simulink model "WL_3_0"  (R2025a)
settings: Solver=ode4  StartTime=0.0  StopTime=T_sim  FixedStep=Dt_sim  RelTol=1e-3
InitFcn:
  | % --- AVVIO AUTOMATICO PYTHON SERVER CON POP-UP (METODO FILE ROBUSTO) ---
  | fprintf('[Simulink] Preparazione simulazione...\n');
  | 
  | % 1. Pop-up per la Raffica
  | scelta_gust = questdlg('Vuoi includere la raffica (gust_H40.gust)?', ...
  |     'Configurazione Raffica', 'Si', 'No', 'No');
  | if isempty(scelta_gust), scelta_gust = 'No'; end
  | 
  | % 2. Pop-up per il Video
  | scelta_video = questdlg('Vuoi generare il video MP4 a fine simulazione?', ...
  |     'Configurazione Video', 'Si', 'No', 'No');
  | if isempty(scelta_video), scelta_video = 'No'; end
  | 
  | % --- PERCORSO ASSOLUTO ---
  | % Definiamo subito la cartella così MATLAB e WSL salvano e leggono dallo stesso posto
  | percorso = '/home/lpmatteo/Internship_INCARBONE_2026/LQR_first_controller_study/LQR_WL_simulation';
  | file_inputs = fullfile(percorso, 'python_inputs.txt');
  | 
  | % --- CREAZIONE FILE DI INPUT ---
  | fid = fopen(file_inputs, 'w');
  | fprintf(fid, '1\n'); % Scelta controller: 1 (LQI)
  | 
  | if strcmp(scelta_gust, 'Si')
  |     fprintf(fid, 's\n');
  | else
  |     fprintf(fid, 'n\n');
  | end
  | 
  | if strcmp(scelta_video, 'Si')
  |     % Se vogliamo il video, precompiliamo anche formato (mp4), qualità (high)
  |     % e la "Y" finale per far partire il render ASWING in automatico.
  |     fprintf(fid, 's\ngif\nmedium\nY\n');
  | else
  |     fprintf(fid, 'n\n');
  | end
  | fclose(fid);
  | 
  | % --- AVVIO DEL SERVER WSL ---
  | % Diciamo a Python di prendere le risposte direttamente dal file appena creato
  | cmd_wsl = sprintf('start "WingLoop Python Server" wsl -e bash -ic "cd %s && conda activate WINGLOOP && python3 controller_wingloop.py < python_inputs.txt; exec bash"', percorso);
  | 
  | system(cmd_wsl);
values from neighbouring files (symbols this model uses):
  u_trim = [0, F2ref, F3ref, 0, E2ref, E2ref]    [WL_main.m]
undefined symbols (not defined in the file or in its folder): FullModel, idx, K_z, matrices, ref_vec
libraries: cstblocks x1
settings Model: SimulationMode=accelerator  Creator=lpmat  LastModifiedBy=lpmat

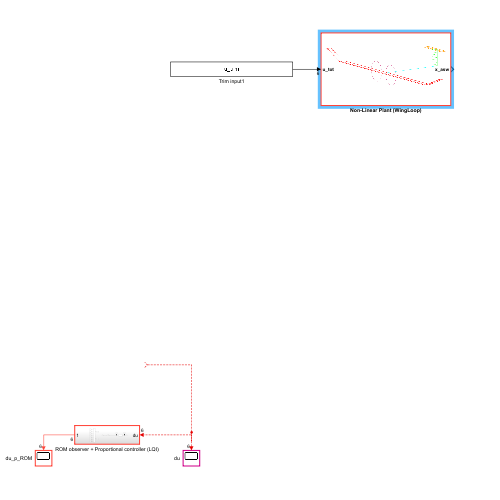
[thumbnail: Simulink's stored preview of the top-level diagram]
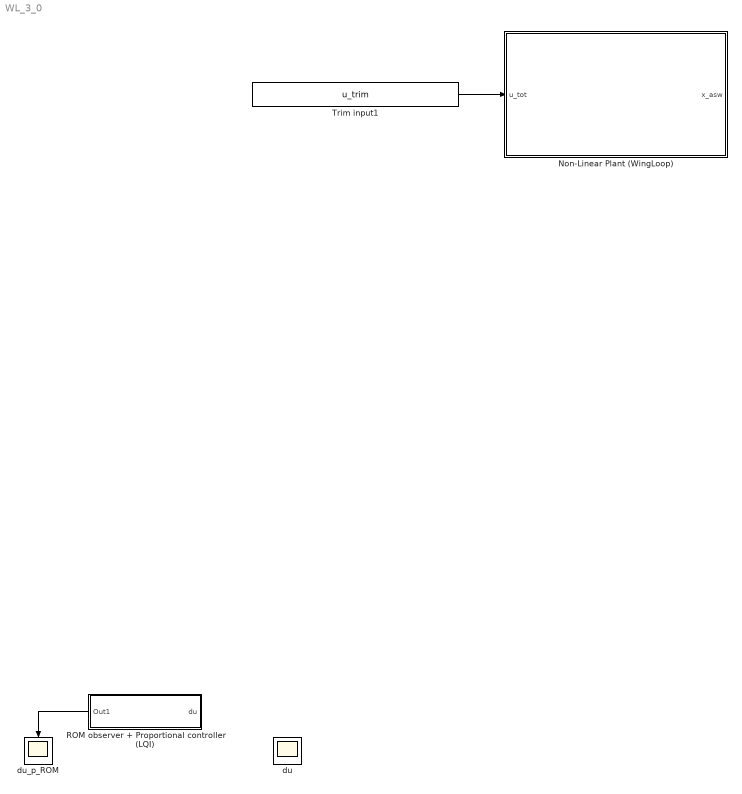
== system WL_3_0 ==
  Non-Linear Plant (WingLoop) : Subsystem
      mask Display: image('Screenshot 2026-03-18 123158.png');
  ROM observer + Proportional controller (LQI) : Subsystem
  Trim input1 : Constant  Value=u_trim
  du : Scope
      settings: ActiveDisplayYMinimum=-1  ActiveDisplayYMaximum=1  DataLoggingVariableName=ScopeData15
  du_p_ROM : Scope
      settings: ActiveDisplayYMinimum=-1  ActiveDisplayYMaximum=1  DataLoggingVariableName=ScopeData10
  wires:
  Trim input1/1 -> Non-Linear Plant (WingLoop)/1(u_tot)
  ROM observer + Proportional controller (LQI)/1(Out1) -> du_p_ROM/1
  ? -> ROM observer + Proportional controller (LQI)/1(du), du/1

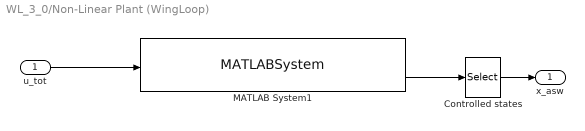
== system WL_3_0/Non-Linear Plant (WingLoop) ==
  u_tot : Inport
  Controlled states : Selector  InputPortWidth=1888  IndexOptions=Index vector (dialog)  Indices=[1:1882]  OutputSizes=1
  MATLAB System1 : MATLABSystem  System=AswingPlant  ServerHost=localhost  ServerPort=5005  NumModalStates=ROM.n_modal  NumPhysicalStates=FullModel.n_orig+ FullModel.n_in  SimulateUsing=Interpreted execution
      mask Type: AswingPlant
  x_asw : Outport
  wires:
  MATLAB System1/2 -> Controlled states/1
  u_tot/1 -> MATLAB System1/1
  Controlled states/1 -> x_asw/1

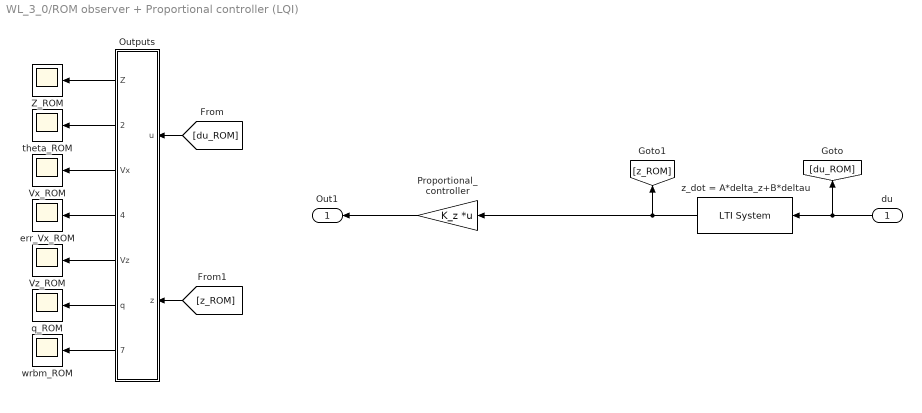
== system WL_3_0/ROM observer + Proportional controller (LQI) ==
  du : Inport
  Outputs : Subsystem
  Proportional_controller : Gain  Gain=K_z  Multiplication=Matrix(K*u)
  Vx_ROM : Scope
      settings: ActiveDisplayYMinimum=-29.75997799121388  ActiveDisplayYMaximum=-29.616858798151441  DataLoggingVariableName=ScopeData28
  Vz_ROM : Scope
      settings: ActiveDisplayYMinimum=-2.6148202510273633  ActiveDisplayYMaximum=-2.6136511943302931  DataLoggingVariableName=ScopeData29
  "Z_ROM " : Scope
      settings: ActiveDisplayYMinimum=-1.6253200350743973E-7  ActiveDisplayYMaximum=1.4627880315669578E-6  DataLoggingVariableName=ScopeData30
  err_Vx_ROM : Scope
      settings: ActiveDisplayYMinimum=-0.016507868182031336  ActiveDisplayYMaximum=0.11294531868689238  DataLoggingVariableName=ScopeData31
  q_ROM : Scope
      settings: ActiveDisplayYMinimum=-0.031623634831333659  ActiveDisplayYMaximum=0.0093452758439209  DataLoggingVariableName=ScopeData32
  theta_ROM : Scope
      settings: ActiveDisplayYMinimum=0.087579549883469346  ActiveDisplayYMaximum=0.088048251339121  DataLoggingVariableName=ScopeData33
  wrbm_ROM : Scope
      settings: ActiveDisplayYMinimum=17.5112693898615  ActiveDisplayYMaximum=17.875639730778097  DataLoggingVariableName=ScopeData34
  z_dot = A*delta_z+B*deltau : cstblocks/LTI System  sys=sys_fb  IC=0  PadeOrder=0
      link override Input Delay: Ts=-1
  Out1 : Outport
  wires:
  du/1 -> z_dot = A*delta_z+B*deltau/1, [du_ROM]
  Outputs/1(Z) -> "Z_ROM "/1
  Outputs/5(Vz) -> Vz_ROM/1
  Outputs/6(q) -> q_ROM/1
  Outputs/3(Vx) -> Vx_ROM/1
  Outputs/4(err_Vx) -> err_Vx_ROM/1
  Outputs/7(wrbm) -> wrbm_ROM/1
  Outputs/2(theta) -> theta_ROM/1
  [du_ROM] -> Outputs/1(u)
  [z_ROM] -> Outputs/2(z)
  Proportional_controller/1 -> Out1/1
  z_dot = A*delta_z+B*deltau/1 -> Proportional_controller/1, [z_ROM]

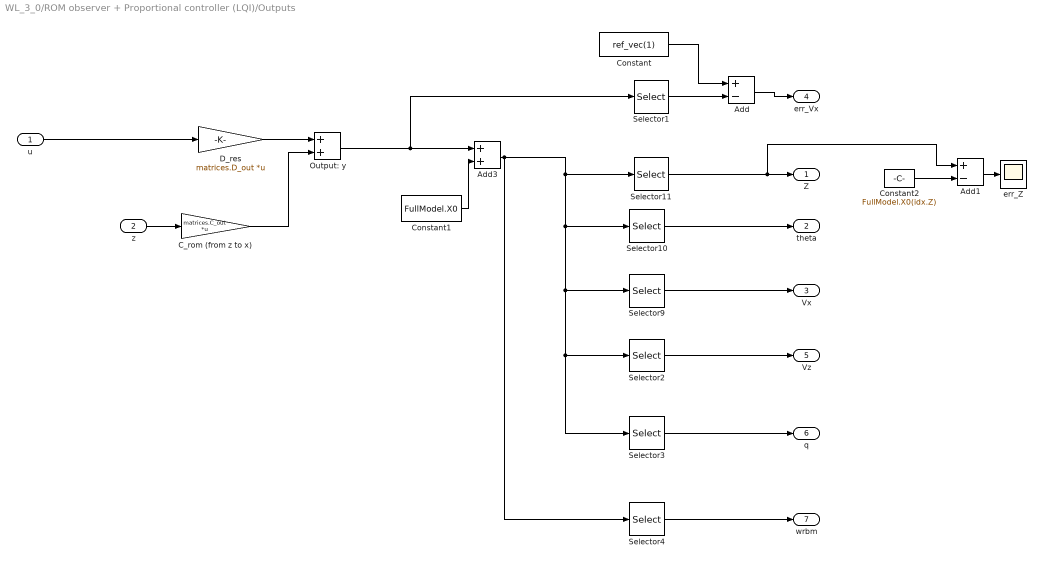
== system WL_3_0/ROM observer + Proportional controller (LQI)/Outputs ==
  u : Inport
  z : Inport  Port=2
  Add : Sum  Inputs=+-
  Add1 : Sum  Inputs=+-
  Add3 : Sum
  C_rom (from z to x) : Gain  Gain=matrices.C_out  Multiplication=Matrix(K*u)
  Constant : Constant  Value=ref_vec(1)
  Constant1 : Constant  Value=FullModel.X0
  Constant2 : Constant  Value=FullModel.X0(idx.Z)
  D_res : Gain  Gain=matrices.D_out  Multiplication=Matrix(K*u)
  Output: y : Sum
  Selector1 : Selector  InputPortWidth=1882  IndexOptions=Index vector (dialog)  Indices=[idx.Vx]  OutputSizes=1
  Selector10 : Selector  InputPortWidth=1882  IndexOptions=Index vector (dialog)  Indices=[idx.theta]  OutputSizes=1
  Selector11 : Selector  InputPortWidth=1882  IndexOptions=Index vector (dialog)  Indices=[idx.Z]  OutputSizes=1
  Selector2 : Selector  InputPortWidth=1882  IndexOptions=Index vector (dialog)  Indices=[idx.Vz]  OutputSizes=1
  Selector3 : Selector  InputPortWidth=1882  IndexOptions=Index vector (dialog)  Indices=[idx.q]  OutputSizes=1
  Selector4 : Selector  InputPortWidth=1882  IndexOptions=Index vector (dialog)  Indices=[idx.wrbm_L]  OutputSizes=1
  Selector9 : Selector  InputPortWidth=1882  IndexOptions=Index vector (dialog)  Indices=[idx.Vx]  OutputSizes=1
  err_Z : Scope
      settings: ActiveDisplayYMinimum=-0.52989229015549089  ActiveDisplayYMaximum=0.058876921128387862  DataLoggingVariableName=ScopeData20
  Z : Outport
  theta : Outport  Port=2
  Vx : Outport  Port=3
  err_Vx : Outport  Port=4
  Vz : Outport  Port=5
  q : Outport  Port=6
  wrbm : Outport  Port=7
  wires:
  C_rom (from z to x)/1 -> Output: y/2
  Constant1/1 -> Add3/2
  D_res/1 -> Output: y/1
  u/1 -> D_res/1
  Output: y/1 -> Selector1/1, Add3/1
  Selector10/1 -> theta/1
  z/1 -> C_rom (from z to x)/1
  Selector9/1 -> Vx/1
  Selector1/1 -> Add/2
  Add/1 -> err_Vx/1
  Constant/1 -> Add/1
  Selector11/1 -> Add1/1, Z/1
  Constant2/1 -> Add1/2
  Add1/1 -> err_Z/1
  Selector2/1 -> Vz/1
  Selector3/1 -> q/1
  Selector4/1 -> wrbm/1
  Add3/1 -> Selector4/1, Selector11/1, Selector10/1, Selector3/1, Selector2/1, Selector9/1
